simulink subsystem "BMS"  (R2023b)
settings: Solver=VariableStepAuto  StartTime=0.0  StopTime=10.0  RelTol=1e-3
libraries: simulink x1
settings Model: Creator=diego  LastModifiedBy=matat

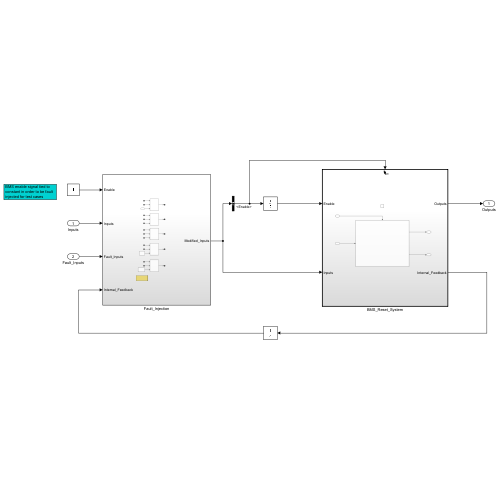
[thumbnail: Simulink's stored preview of the top-level diagram]
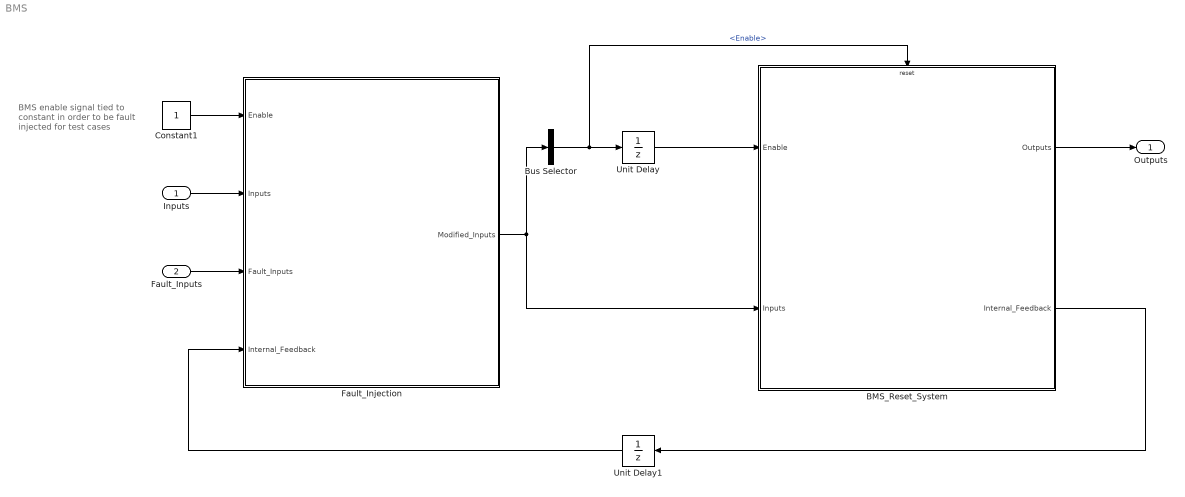
== system BMS ==
  note: BMS enable signal tied to constant in order to be fault injected for test cases
  Inputs : Inport
  Fault_Inputs : Inport  Port=2
  "BMS_Reset_System " : Subsystem  TreatAsAtomicUnit=on
  Bus Selector : BusSelector  OutputSignals=Enable
  Constant1 : Constant
  Fault_Injection : Subsystem
  Unit Delay : UnitDelay  SampleTime=-1  HasFrameUpgradeWarning=on
  Unit Delay1 : UnitDelay  SampleTime=-1  HasFrameUpgradeWarning=on
  Outputs : Outport
  wires:
  "BMS_Reset_System "/1(Outputs) -> Outputs/1
  Fault_Injection/1(Modified_Inputs) -> "BMS_Reset_System "/2(Inputs), Bus Selector/1
  Unit Delay/1 -> "BMS_Reset_System "/1(Enable)
  Constant1/1 -> Fault_Injection/1(Enable)
  Inputs/1 -> Fault_Injection/2(Inputs)
  Fault_Inputs/1 -> Fault_Injection/3(Fault_Inputs)
  "BMS_Reset_System "/2(Internal_Feedback) -> Unit Delay1/1
  Unit Delay1/1 -> Fault_Injection/4(Internal_Feedback)
  Bus Selector/1 -> Unit Delay/1, "BMS_Reset_System "/Reset  "<Enable>"

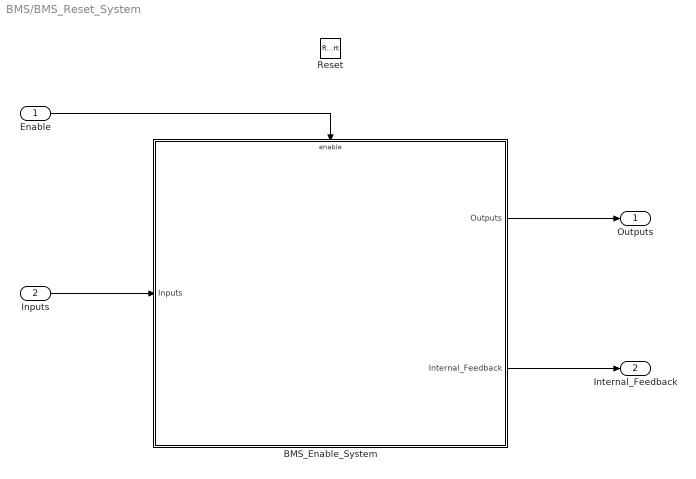
== system BMS/BMS_Reset_System  ==
  Enable : Inport
  Inputs : Inport  Port=2
  Reset : ResetPort  DisableCoverage=on  ResetTriggerType=falling
  "BMS_Enable_System " : Subsystem  TreatAsAtomicUnit=on
  Outputs : Outport
  Internal_Feedback : Outport  Port=2
  wires:
  Inputs/1 -> "BMS_Enable_System "/1(Inputs)
  "BMS_Enable_System "/1(Outputs) -> Outputs/1
  Enable/1 -> "BMS_Enable_System "/Enable
  "BMS_Enable_System "/2(Internal_Feedback) -> Internal_Feedback/1

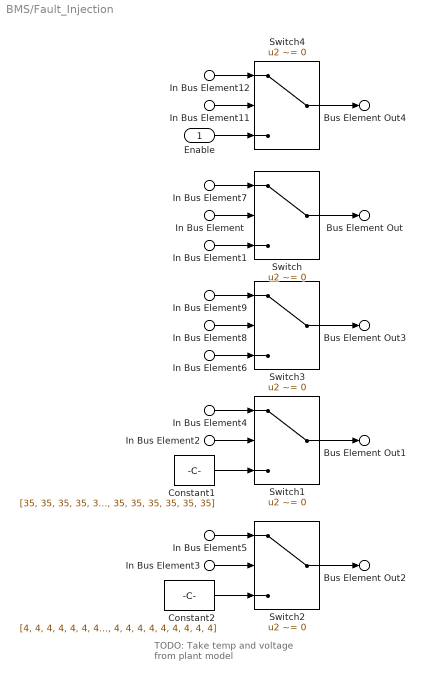
== system BMS/Fault_Injection ==
  note: TODO: Take temp and voltage from plant model
  Enable : Inport
  In Bus Element1 : Inport  Port=2  PortName=Inputs  Element=VCU_Outputs.BMS_Contactor_Command
  In Bus Element : Inport  Port=3  PortName=Fault_Inputs  Element=Override_BMS_Contactor_State
  In Bus Element2 : Inport  Port=3  PortName=Fault_Inputs  Element=Override_Cell_Temps
  In Bus Element3 : Inport  Port=3  PortName=Fault_Inputs  Element=Override_Cell_Voltages
  In Bus Element4 : Inport  Port=3  PortName=Fault_Inputs  Element=Cell_Temps
  In Bus Element5 : Inport  Port=3  PortName=Fault_Inputs  Element=Cell_Voltages
  In Bus Element7 : Inport  Port=3  PortName=Fault_Inputs  Element=BMS_Contactor_State
  In Bus Element8 : Inport  Port=3  PortName=Fault_Inputs  Element=Override_BMS_Previous_State
  In Bus Element9 : Inport  Port=3  PortName=Fault_Inputs  Element=BMS_Previous_State
  In Bus Element12 : Inport  Port=3  PortName=Fault_Inputs  Element=BMS_EN
  In Bus Element11 : Inport  Port=3  PortName=Fault_Inputs  Element=Override_BMS_EN
  In Bus Element6 : Inport  Port=4  PortName=Internal_Feedback  Element=Contactor_Closed
  Constant1 : Constant  Value=[35, 35, 35, 35, 35, 35, 35, 35, 35, 35, 35, 35, 35, 35, 35, 35, 35, 35, 35, 35, 35, 35, 35, 35, 35, 35, 35, 35, 35, 35, 35, 35, 35, 35, 35, 35, 35, 35, 35, 35, 35, 35, 35, 35, 35]
  Constant2 : Constant  Value=[4, 4, 4, 4, 4, 4, 4, 4, 4, 4, 4, 4, 4, 4, 4, 4, 4, 4, 4, 4, 4, 4, 4, 4, 4, 4, 4, 4, 4, 4, 4, 4, 4, 4, 4, 4, 4, 4, 4, 4, 4, 4, 4, 4, 4, 4, 4, 4, 4, 4, 4, 4, 4, 4, 4, 4, 4, 4, 4, 4, 4, 4, 4, 4, 4, 4, 4, 4, 4, 4, 4, 4, 4, 4, 4, 4, 4, 4, 4, 4, 4, 4, 4, 4, 4, 4, 4, 4, 4, 4, 4, 4, 4, 4, 4, 4, 4, 4, 4, 4]
  Switch{,1..4} (5 alike) : Switch  Criteria=u2 ~= 0  SaturateOnIntegerOverflow=off  InputSameDT=off
  Bus Element Out : Outport  PortName=Modified_Inputs  Element=VCU_Inputs.BMS_Contactor_Command
  Bus Element Out1 : Outport  PortName=Modified_Inputs  Element=Cell_Temps
  Bus Element Out2 : Outport  PortName=Modified_Inputs  Element=Cell_Voltages
  Bus Element Out3 : Outport  PortName=Modified_Inputs  Element=Contactor_Closed
  Bus Element Out4 : Outport  PortName=Modified_Inputs  Element=Enable
  wires:
  Switch/1 -> Bus Element Out/1
  In Bus Element5/1 -> Switch2/1
  Switch1/1 -> Bus Element Out1/1
  In Bus Element7/1 -> Switch/1
  In Bus Element/1 -> Switch/2
  In Bus Element1/1 -> Switch/3
  In Bus Element2/1 -> Switch1/2
  Constant2/1 -> Switch2/3
  Constant1/1 -> Switch1/3
  In Bus Element3/1 -> Switch2/2
  Switch2/1 -> Bus Element Out2/1
  In Bus Element4/1 -> Switch1/1
  In Bus Element6/1 -> Switch3/3
  Switch3/1 -> Bus Element Out3/1
  In Bus Element9/1 -> Switch3/1
  In Bus Element8/1 -> Switch3/2
  In Bus Element11/1 -> Switch4/2
  Enable/1 -> Switch4/3
  Switch4/1 -> Bus Element Out4/1
  In Bus Element12/1 -> Switch4/1

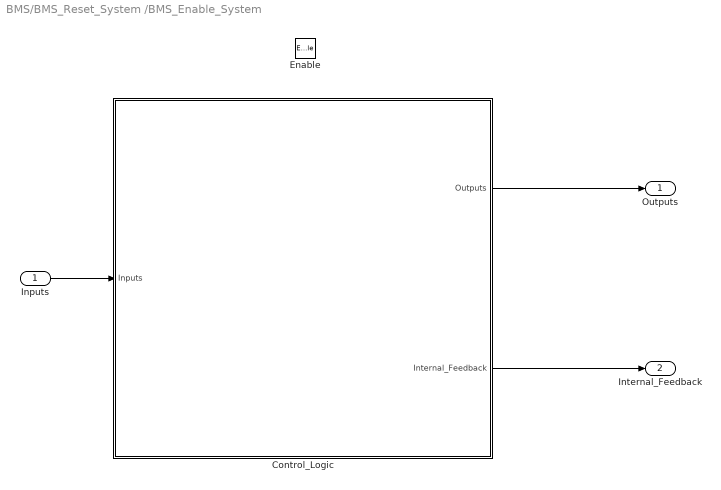
== system BMS/BMS_Reset_System /BMS_Enable_System  ==
  Inputs : Inport
  Enable : EnablePort  StatesWhenEnabling=reset
  Control_Logic : Subsystem
  Outputs : Outport
  Internal_Feedback : Outport  Port=2
  wires:
  Control_Logic/1(Outputs) -> Outputs/1
  Inputs/1 -> Control_Logic/1(Inputs)
  Control_Logic/2(Internal_Feedback) -> Internal_Feedback/1

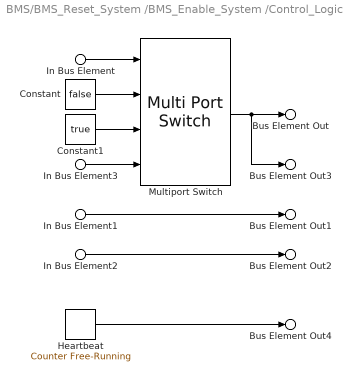
== system BMS/BMS_Reset_System /BMS_Enable_System /Control_Logic ==
  In Bus Element : Inport  PortName=Inputs  Element=VCU_Inputs.BMS_Contactor_Command
  In Bus Element1 : Inport  PortName=Inputs  Element=Cell_Temps
  In Bus Element2 : Inport  PortName=Inputs  Element=Cell_Voltages
  In Bus Element3 : Inport  PortName=Inputs  Element=Contactor_Closed
  Constant : Constant  Value=false
  Constant1 : Constant  Value=true
  Heartbeat : simulink/Sources/Counter Free-Running  NumBits=32  tsamp=-1
  Multiport Switch : MultiPortSwitch  DataPortOrder=Specify indices  DataPortIndices={BMS_Contactor_Command.Open_Contactor, BMS_Contactor_Command.Close_Contactor, BMS_Contactor_Command.Stay}  SaturateOnIntegerOverflow=off  InputSameDT=off
  Bus Element Out : Outport  PortName=Outputs  Element=BMS_Feedback.Contactor_Closed
  Bus Element Out1 : Outport  PortName=Outputs  Element=BMS_Feedback.Cell_Temps
  Bus Element Out2 : Outport  PortName=Outputs  Element=BMS_Feedback.Cell_Voltages
  Bus Element Out4 : Outport  PortName=Outputs  Element=BMS_Feedback.BMS_Heartbeat
  Bus Element Out3 : Outport  Port=2  PortName=Internal_Feedback  Element=Contactor_Closed
  wires:
  Heartbeat/1 -> Bus Element Out4/1
  In Bus Element1/1 -> Bus Element Out1/1
  In Bus Element2/1 -> Bus Element Out2/1
  In Bus Element/1 -> Multiport Switch/1
  Constant/1 -> Multiport Switch/2
  Constant1/1 -> Multiport Switch/3
  Multiport Switch/1 -> Bus Element Out/1, Bus Element Out3/1
  In Bus Element3/1 -> Multiport Switch/4
